simulink model "thermal_control_block"  (Simulink 7.3)
settings: Solver=ode45  StartTime=0.0  StopTime=10.0  RelTol=1e-3
undefined symbols (not defined in the file): Gam, H, J, Phi, Rth_max
settings Model: Creator=Administrator  LastModifiedBy=Administrator

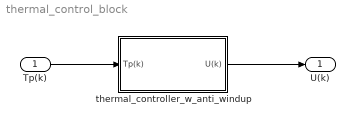
== system thermal_control_block ==
  Tp(k) : Inport  PortDimensions=1  DataType=double  OutDataTypeStr=double
  thermal_controller_w_anti_windup : Subsystem  mask{kp=38.6, kp_max=400, kp_min=0, Rth=0.467, Cth=295.7, Pidle=13.3, Ts=10, Ts_u=1, Umin=0.1, Umax=0.67, To=20, Tmax=70}
      mask prompts: kp "Enter Plant Gain [kp]"; kp_max "Enter Plant Gain Max [kp_max]"; kp_min "Enter Plant Gain Min [kp_min]"; Rth "Enter Thermal Resistance [Rth]"; Cth "Enter Thermal Capacitance [Cth]"; Pidle "Idle Power [Pidle]"; Ts "Digital Controller Sample Rate [Ts]"; Ts_u "Simulated Model Sample Rate [Ts_u]"; To "Room Temperature [To]"; Tmax "Max Processor Temperature [Tmax]"
  U(k) : Outport
  wires:
  thermal_controller_w_anti_windup/1(U(k)) -> U(k)/1
  Tp(k)/1 -> thermal_controller_w_anti_windup/1(Tp(k))

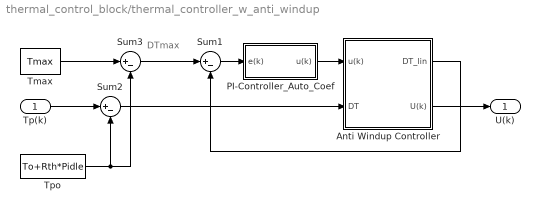
== system thermal_control_block/thermal_controller_w_anti_windup ==
  note: DTmax
  Tp(k) : Inport  PortDimensions=1  DataType=double  OutDataTypeStr=double
  Anti Windup Controller : Subsystem  mask{kp=kp, kp_max=kp_max, kp_min=kp_min, Rth=Rth, Cth=Cth, Ts=Ts, Ts_u=Ts_u, Umin=Umin, Umax=Umax}
      mask prompts: kp "Enter Plant Gain [kp]"; kp_max "Enter Plant Gain Max [kp_max]"; kp_min "Enter Plant Gain Min [kp_min]"; Rth "Enter thermal Resistance [Rth]"; Cth "Enter Thermal Capacitance [Cth]"; Ts "Digital Controller Sample Rate [Ts]"; Ts_u "Simulated Model Sample Rate [Ts_u]"
  PI-Controller_Auto_Coef : Subsystem  mask{kp_max=kp_max, Rth_max=Rth_max, Cth=Cth, GM=3, Ts=Ts, kp=kp, Rth=Rth}
      mask prompts: kp_max "Enter kp_max [kp_max]"; Rth_max "Enter Rth_max [Rth_max]"; Cth "Enter Cth [Cth]"; GM "Enter desired gain margin (dB) [GM]"; Ts "Enter Sample Time (s) [Ts]"; kp "Enter kp [kp]"; Rth "Enter Rth [Rth]"
      mask init:
      | k_GM=10^(-GM/20)
      | [Phi,Gam,H,J,Ts]=mpc_dt_model(kp,Rth,Cth,Ts);
      | [Phi_max,Gam_max,H,J,Ts]=mpc_dt_model(kp_max,Rth_max,Cth,Ts);
      | Phi
      | Phi_max
      | Gam
      | Gam_max
      | wi=2*(1-Phi_max)/(Ts*(1+Phi_max))
      | Kp=k_GM*(1+Phi_max)/(2*Gam_max)
      | Ki=2*k_GM/(Gam_max*(2+wi*Ts))
      | Hpz_wc=tf(Gam_max,[1,-Phi_max],Ts)
      | Hpz=tf(Gam,[1,-Phi],Ts)
      | Hsi=tf(Ki*[1,wi],[1,0])
      | Kzi=ipesh_transform(Hsi,Ts)
      | Kz=Kp+Kzi
  Sum1 : Sum  Inputs=|+-  OutDataType=sfix(16)  OutScaling=2^0
  Sum2 : Sum  Inputs=|+-  OutDataType=sfix(16)  OutScaling=2^0
  Sum3 : Sum  Inputs=|+-  OutDataType=sfix(16)  OutScaling=2^0
  Tmax : Constant  Value=Tmax  OutDataType=sfix(16)  OutScaling=2^0  SampleTime=-1
  Tpo : Constant  Value=To+Rth*Pidle  OutDataType=sfix(16)  OutScaling=2^0  SampleTime=-1
  U(k) : Outport
  wires:
  PI-Controller_Auto_Coef/1(u(k)) -> Anti Windup Controller/1(u(k))
  Anti Windup Controller/1(DT_lin) -> Sum1/2
  Anti Windup Controller/2(U(k)) -> U(k)/1
  Sum1/1 -> PI-Controller_Auto_Coef/1(e(k))
  Tp(k)/1 -> Sum2/1
  Tpo/1 -> Sum2/2, Sum3/2
  Sum2/1 -> Anti Windup Controller/2(DT)
  Tmax/1 -> Sum3/1
  Sum3/1 -> Sum1/1

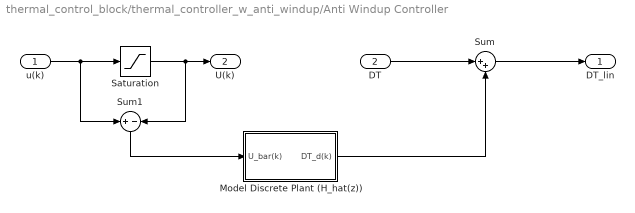
== system thermal_control_block/thermal_controller_w_anti_windup/Anti Windup Controller ==
  u(k) : Inport
  DT : Inport  Port=2
  Model Discrete Plant (H_hat(z)) : Subsystem  mask{kp=kp, Rth=Rth, Cth=Cth, Ts=Ts, Umin=Umin}
      mask prompts: kp "Enter Plant Gain [kp]"; Rth "Enter Thermal Resistance [Rth]"; Cth "Enter Thermal Capacitance [Cth]"; Ts "Enter Sample Rate (seconds) [Ts]"; Umin "Enter Umin"
      mask init:
      | [Phi,Gam,H,J,Ts]=mpc_dt_model(kp,Rth,Cth,Ts);
      | X0=0*kp*Rth;
      | Gzoh=ss(Phi,Gam,H,J,Ts);
  Saturation : Saturate  UpperLimit=Umax  LowerLimit=Umin  ZeroCross=off  OutDataType=sfix(16)  OutScaling=2^0
  Sum : Sum  Inputs=|++  OutDataType=sfix(16)  OutScaling=2^0
  Sum1 : Sum  Inputs=+|-  OutDataType=sfix(16)  OutScaling=2^0
  DT_lin : Outport
  U(k) : Outport  Port=2
  wires:
  DT/1 -> Sum/1
  Sum/1 -> DT_lin/1
  Model Discrete Plant (H_hat(z))/1(DT_d(k)) -> Sum/2
  Sum1/1 -> Model Discrete Plant (H_hat(z))/1(U_bar(k))
  u(k)/1 -> Sum1/1, Saturation/1
  Saturation/1 -> U(k)/1, Sum1/2

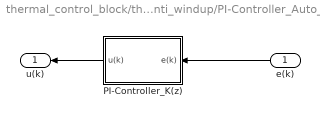
== system thermal_control_block/thermal_controller_w_anti_windup/PI-Controller_Auto_Coef ==
  e(k) : Inport
  PI-Controller_K(z) : Subsystem  mask{Kp=Kp, Ki=Ki, wi=wi, Ts=Ts}
      mask prompts: Kp "Enter Proportional Gain [Kp]"; Ki "Enter Integral Gain [Ki]"; wi "Enter Integral Omega (rad/s) [wi]"; Ts "Enter Sample Time (s) [Ts]"
  u(k) : Outport
  wires:
  PI-Controller_K(z)/1(u(k)) -> u(k)/1
  e(k)/1 -> PI-Controller_K(z)/1(e(k))

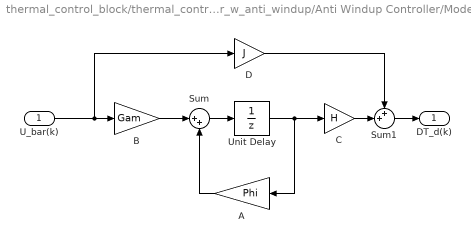
== system thermal_control_block/thermal_controller_w_anti_windup/Anti Windup Controller/Model Discrete Plant (H_hat(z)) ==
  U_bar(k) : Inport
  A : Gain  Gain=Phi  ParameterDataType=fixdt(1, 16)  ParameterScaling=2^0  OutDataType=fixdt(1, 16)  OutScaling=2^0
  B : Gain  Gain=Gam  ParameterDataType=fixdt(1, 16)  ParameterScaling=2^0  OutDataType=fixdt(1, 16)  OutScaling=2^0
  C : Gain  Gain=H  ParameterDataType=fixdt(1, 16)  ParameterScaling=2^0  OutDataType=fixdt(1, 16)  OutScaling=2^0
  D : Gain  Gain=J  ParameterDataType=fixdt(1, 16)  ParameterScaling=2^0  OutDataType=fixdt(1, 16)  OutScaling=2^0
  Sum : Sum  Inputs=|++  OutDataType=fixdt(1, 16)  OutScaling=2^0
  Sum1 : Sum  Inputs=++|  OutDataType=fixdt(1, 16)  OutScaling=2^0
  Unit Delay : UnitDelay  X0=X0  SampleTime=-1
  DT_d(k) : Outport
  wires:
  Unit Delay/1 -> C/1, A/1
  D/1 -> Sum1/1
  C/1 -> Sum1/2
  Sum1/1 -> DT_d(k)/1
  U_bar(k)/1 -> D/1, B/1
  B/1 -> Sum/1
  Sum/1 -> Unit Delay/1
  A/1 -> Sum/2

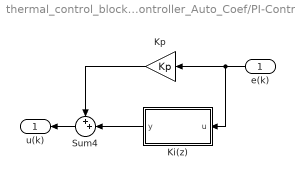
== system thermal_control_block/thermal_controller_w_anti_windup/PI-Controller_Auto_Coef/PI-Controller_K(z) ==
  e(k) : Inport
  Ki(z) : Subsystem  mask{num=Ki*[1,wi], den=[1,0], Ts=Ts}
      mask prompts: num "Enter num of H(s) [num]"; den "Enter den of H(s) [den]"; Ts "Enter sample time (s) [Ts]"
      mask init:
      | Hs=tf(num,den);
      | Hz=ipesh_transform(Hs,Ts);
  Kp : Gain  Gain=Kp  ParameterDataType=sfix(16)  ParameterScaling=2^0  OutDataType=sfix(16)  OutScaling=2^0
  Sum4 : Sum  Inputs=++|  OutDataType=sfix(16)  OutScaling=2^0
  u(k) : Outport
  wires:
  Sum4/1 -> u(k)/1
  Kp/1 -> Sum4/1
  Ki(z)/1(y) -> Sum4/2
  e(k)/1 -> Ki(z)/1(u), Kp/1

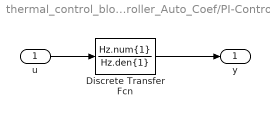
== system thermal_control_block/thermal_controller_w_anti_windup/PI-Controller_Auto_Coef/PI-Controller_K(z)/Ki(z) ==
  u : Inport
  Discrete Transfer Fcn : DiscreteTransferFcn  Numerator=Hz.num{1}  Denominator=Hz.den{1}  SampleTime=Ts
  y : Outport
  wires:
  Discrete Transfer Fcn/1 -> y/1
  u/1 -> Discrete Transfer Fcn/1
